simulink subsystem "GS3DX_KDS_Spherical"  (R2025b)
settings: Solver=VariableStepAuto  StartTime=0.0  StopTime=10.0  RelTol=1e-3
model mask{StartPositionX=0, StartPositionY=0, StartPositionZ=0, StartVelocityX=0, StartVelocityY=0, StartVelocityZ=0, DampeningX=0, DampeningY=0, DampeningZ=0, RxPositionTargetPriority=None, RyPositionTargetPriority=None, RzPositionTargetPriority=None, RxVelocityTargetPriority=None, RyVelocityTargetPriority=None, RzVelocityTargetPriority=None}
  mask prompts: StartPositionX "Start Position X (deg)"; StartPositionY "Start Position Y (deg)"; StartPositionZ "Start Position Z (deg)"; StartVelocityX "Start Velocity X (deg/s)"; StartVelocityY "Start Velocity Y (deg/s)"; StartVelocityZ "Start Velocity Z (deg/s)"; DampeningX "Dampening X (Nm/deg/s)"; DampeningY "Dampening Y (Nm/deg/s)"; DampeningZ "Dampening Z (Nm/deg/s)"; RxPositionTargetPriority "Position Target Priority X"; RyPositionTargetPriority "Position Target Priority Y"; RzPositionTargetPriority "Position Target Priority Z"; RxVelocityTargetPriority "Velocity Target Priority X"; RyVelocityTargetPriority "Velocity Target Priority Y"; RzVelocityTargetPriority "Velocity Target Priority Z"
undefined symbols (not defined in the file): DampeningGlobalGain, gs3dx_xyz_rate_matrix, LocalDampeningEnable, X, Y, Z
libraries: nesl_utility x13, sm_lib x3
settings Model: Creator=diete  LastModifiedBy=diete

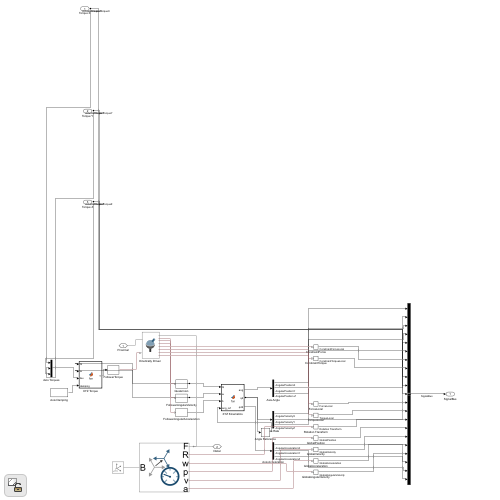
[thumbnail: Simulink's stored preview of the top-level diagram]
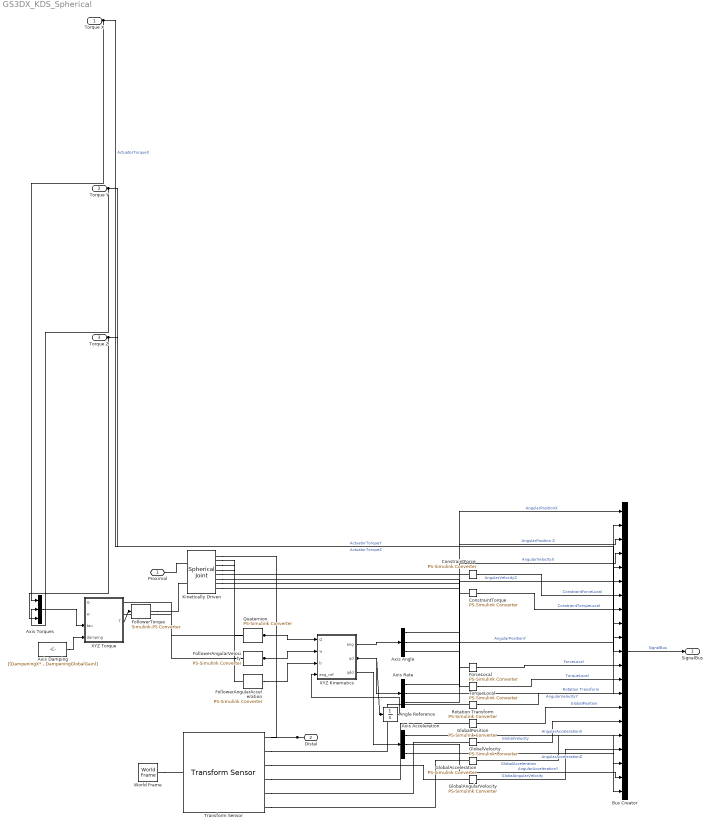
== system GS3DX_KDS_Spherical ==
  Torque X : Inport
  Torque Y : Inport  Port=2
  Torque Z : Inport  Port=3
  Angle Reference : Integrator  InitialCondition=[(StartPositionX); (StartPositionY); (StartPositionZ)]
  Axis Acceleration : Demux  Outputs=3
  Axis Angle : Demux  Outputs=3
  Axis Damping : Constant  Value=[(DampeningX*LocalDampeningEnable*DampeningGlobalGain); (DampeningY*LocalDampeningEnable*DampeningGlobalGain); (DampeningZ*LocalDampeningEnable*DampeningGlobalGain)]  SampleTime=0
  Axis Rate : Demux  Outputs=3
  Axis Torques : Mux  Inputs=3
  Bus Creator : BusCreator  Inputs=21
  ConstraintForce : nesl_utility/PS-Simulink Converter  PhysicalDomain=network_engine_domain  SubClassName=ps_output  LeftPortType=input  RightPortType=output  PseudoPeriodic=off  Frequencies=[]  VectorFormat=1-D array  Unit=inherit  AffineConversion=off
  ConstraintTorque : nesl_utility/PS-Simulink Converter  PhysicalDomain=network_engine_domain  SubClassName=ps_output  LeftPortType=input  RightPortType=output  PseudoPeriodic=off  Frequencies=[]  VectorFormat=1-D array  Unit=inherit  AffineConversion=off
  FollowerAngularAcceleration : nesl_utility/PS-Simulink Converter  PhysicalDomain=network_engine_domain  SubClassName=ps_output  LeftPortType=input  RightPortType=output  PseudoPeriodic=off  Frequencies=[]  VectorFormat=inherit  Unit=rad/s^2  AffineConversion=off
  FollowerAngularVelocity : nesl_utility/PS-Simulink Converter  PhysicalDomain=network_engine_domain  SubClassName=ps_output  LeftPortType=input  RightPortType=output  PseudoPeriodic=off  Frequencies=[]  VectorFormat=inherit  Unit=rad/s  AffineConversion=off
  FollowerTorque : nesl_utility/Simulink-PS Converter  PhysicalDomain=network_engine_domain  SubClassName=ps_input  LeftPortType=input  RightPortType=output  PseudoPeriodic=off  Frequencies=[]  NoiseDistribution=none  NoiseParameters=[]  Unit=N*m  AffineConversion=off  FilteringAndDerivatives=provide  SimscapeFilterOrder=1  InputFilterTimeConstant=0.001  UdotUserProvided=0
  ForceLocal : nesl_utility/PS-Simulink Converter  PhysicalDomain=network_engine_domain  SubClassName=ps_output  LeftPortType=input  RightPortType=output  PseudoPeriodic=off  Frequencies=[]  VectorFormat=1-D array  Unit=inherit  AffineConversion=off
  GlobalAcceleration : nesl_utility/PS-Simulink Converter  PhysicalDomain=network_engine_domain  SubClassName=ps_output  LeftPortType=input  RightPortType=output  PseudoPeriodic=off  Frequencies=[]  VectorFormat=1-D array  Unit=inherit  AffineConversion=off
  GlobalAngularVelocity : nesl_utility/PS-Simulink Converter  PhysicalDomain=network_engine_domain  SubClassName=ps_output  LeftPortType=input  RightPortType=output  PseudoPeriodic=off  Frequencies=[]  VectorFormat=1-D array  Unit=deg/s  AffineConversion=off
  GlobalPosition : nesl_utility/PS-Simulink Converter  PhysicalDomain=network_engine_domain  SubClassName=ps_output  LeftPortType=input  RightPortType=output  PseudoPeriodic=off  Frequencies=[]  VectorFormat=1-D array  Unit=inherit  AffineConversion=off
  GlobalVelocity : nesl_utility/PS-Simulink Converter  PhysicalDomain=network_engine_domain  SubClassName=ps_output  LeftPortType=input  RightPortType=output  PseudoPeriodic=off  Frequencies=[]  VectorFormat=1-D array  Unit=inherit  AffineConversion=off
  Kinetically Driven : sm_lib/Joints/Spherical Joint  JointMode=Normal  CompositeWrenchDir=BaseOnFollower  CompositeWrenchFrame=FollowerFrame  SenseConstraintForce=on  SenseConstraintTorque=on  SenseTotalForce=on  SenseTotalTorque=on  PositionTargetSpecify=off  PositionTargetPriority=High  PositionTargetRotationMethod=RotationSequence  PositionTargetFollAlignAxisA=+X  PositionTargetBaseAlignAxisA=+Y  PositionTargetFollAlignAxisB=+Y  PositionTargetBaseAlignAxisB=+Z  PositionTargetRotationStandardAxis=+Z  PositionTargetRotationAngle=0  PositionTargetRotationAngleUnits=deg  PositionTargetRotationArbitraryAxis=[0 0 1]  PositionTargetRotationSequenceAxes=FollowerAxes  PositionTargetRotationSequence=XYZ  PositionTargetRotationSequenceAngles=[(StartPositionX) (StartPositionY) (StartPositionZ)]  PositionTargetRotationSequenceAnglesUnits=deg  PositionTargetRotationMatrix=[1 0 0;0 1 0;0 0 1]  PositionTargetQuaternion=[1 0 0 0]  VelocityTargetSpecify=off  VelocityTargetPriority=High  VelocityTargetValue=gs3dx_xyz_rate_matrix((StartPositionY)*pi/180, (StartPositionZ)*pi/180)*[(StartVelocityX); (StartVelocityY); (StartVelocityZ)]  VelocityTargetValueUnits=deg/s  VelocityTargetInFollowerFrame=on  EqPosRotationMethod=None  EqPosFollAlignAxisA=+X  EqPosBaseAlignAxisA=+Y  EqPosFollAlignAxisB=+Y  EqPosBaseAlignAxisB=+Z  EqPosRotationStandardAxis=+Z  EqPosRotationAngle=0  EqPosRotationAngleUnits=deg  EqPosRotationArbitraryAxis=[0 0 1]  EqPosRotationSequenceAxes=FollowerAxes  EqPosRotationSequence=XYX  EqPosRotationSequenceAngles=[0 0 0]  EqPosRotationSequenceAnglesUnits=deg  EqPosRotationMatrix=[1 0 0;0 1 0;0 0 1]  EqPosQuaternion=[1 0 0 0]  SpringStiffness=0  SpringStiffnessUnits=N*m/deg  DampingCoefficient=0  DampingCoefficientUnits=N*m/(deg/s)  LowerLimitSpecify=off  LowerLimitBound=15  LowerLimitBoundUnits=deg  LowerLimitStiffness=1e4  LowerLimitStiffnessUnits=N*m/deg  LowerLimitDamping=10  LowerLimitDampingUnits=N*m/(deg/s)  LowerLimitTransitionRegionWidth=0.1  LowerLimitTransitionRegionWidthUnits=deg  UpperLimitSpecify=off  UpperLimitBound=45  UpperLimitBoundUnits=deg  UpperLimitStiffness=1e4  UpperLimitStiffnessUnits=N*m/deg  UpperLimitDamping=10  UpperLimitDampingUnits=N*m/(deg/s)  UpperLimitTransitionRegionWidth=0.1  UpperLimitTransitionRegionWidthUnits=deg  TorqueActuationMode=InputTorque  ActuateTorqueX=off  ActuateTorqueY=off  ActuateTorqueZ=off  ActuateTorque=on  ActuationFrame=FollowerFrame  SensePosition=on  SenseVelocityX=off  SenseVelocityY=off  SenseVelocityZ=off  SenseVelocity=on  SenseAccelerationX=off  SenseAccelerationY=off  SenseAccelerationZ=off  SenseAcceleration=on  SenseLowerLimitTorqueMag=off  SenseUpperLimitTorqueMag=off  SensingFrame=FollowerFrame
  Quaternion : nesl_utility/PS-Simulink Converter  PhysicalDomain=network_engine_domain  SubClassName=ps_output  LeftPortType=input  RightPortType=output  PseudoPeriodic=off  Frequencies=[]  VectorFormat=inherit  Unit=1  AffineConversion=off
  Rotation Transform : nesl_utility/PS-Simulink Converter  PhysicalDomain=network_engine_domain  SubClassName=ps_output  LeftPortType=input  RightPortType=output  PseudoPeriodic=off  Frequencies=[]  VectorFormat=1-D array  Unit=inherit  AffineConversion=off
  TorqueLocal : nesl_utility/PS-Simulink Converter  PhysicalDomain=network_engine_domain  SubClassName=ps_output  LeftPortType=input  RightPortType=output  PseudoPeriodic=off  Frequencies=[]  VectorFormat=1-D array  Unit=inherit  AffineConversion=off
  Transform Sensor : sm_lib/Frames and Transforms/Transform Sensor  MeasurementFrame=World  RotationSequence=XYX  SenseAngle=off  SenseAxis=off  SenseQ=off  SenseR=on  SenseRotationSequence=off  SenseOmegaX=off  SenseOmegaY=off  SenseOmegaZ=off  SenseOmega=on  SenseQDot=off  SenseRDot=off  SenseRotationSequenceDot=off  SenseAlphaX=off  SenseAlphaY=off  SenseAlphaZ=off  SenseAlpha=off  SenseQDDot=off  SenseRDDot=off  SenseX=off  SenseY=off  SenseZ=off  SenseXYZ=on  SenseRad=off  SenseAzim=off  SenseDist=off  SenseInc=off  SenseXDot=off  SenseYDot=off  SenseZDot=off  SenseXYZDot=on  SenseRadDot=off  SenseAzimDot=off  SenseDistDot=off  SenseIncDot=off  SenseXDDot=off  SenseYDDot=off  SenseZDDot=off  SenseXYZDDot=on  SenseRadDDot=off  SenseAzimDDot=off  SenseDistDDot=off  SenseIncDDot=off
  World Frame : sm_lib/Frames and Transforms/World Frame
  XYZ Kinematics : MATLAB Function  TreatAsAtomicUnit=on
  XYZ Torque : MATLAB Function  TreatAsAtomicUnit=on
  Proximal : PMIOPort  Side=Left
  Distal : PMIOPort  Port=2  Side=Right
  SignalBus : Outport
  wires:
  Rotation Transform/1 -> Bus Creator/14  "Rotation Transform"
  ForceLocal/1 -> Bus Creator/12  "ForceLocal"
  ConstraintTorque/1 -> Bus Creator/8  "ConstraintTorqueLocal"
  GlobalAcceleration/1 -> Bus Creator/17  "GlobalAcceleration"
  GlobalAngularVelocity/1 -> Bus Creator/18  "GlobalAngularVelocity"
  ConstraintForce/1 -> Bus Creator/7  "ConstraintForceLocal"
  TorqueLocal/1 -> Bus Creator/13  "TorqueLocal"
  GlobalVelocity/1 -> Bus Creator/16  "GlobalVelocity"
  GlobalPosition/1 -> Bus Creator/15  "GlobalPosition"
  Bus Creator/1 -> SignalBus/1  "SignalBus"
  Torque X/1 -> Axis Torques/1, Bus Creator/9  "ActuatorTorqueX"
  Torque Y/1 -> Axis Torques/2, Bus Creator/10  "ActuatorTorqueY"
  Torque Z/1 -> Axis Torques/3, Bus Creator/11  "ActuatorTorqueZ"
  Quaternion/1 -> XYZ Torque/1(Q), XYZ Kinematics/1(Q)
  FollowerAngularVelocity/1 -> XYZ Torque/2(w), XYZ Kinematics/2(w)
  Axis Torques/1 -> XYZ Torque/3(tau)
  Axis Damping/1 -> XYZ Torque/4(damping)
  XYZ Torque/1(T) -> FollowerTorque/1
  FollowerAngularAcceleration/1 -> XYZ Kinematics/3(b)
  Angle Reference/1 -> XYZ Kinematics/4(ang_ref)
  XYZ Kinematics/2(qd) -> Angle Reference/1, Axis Rate/1
  XYZ Kinematics/1(ang) -> Axis Angle/1
  Axis Angle/1 -> Bus Creator/1  "AngularPositionX"
  Axis Angle/2 -> Bus Creator/2  "AngularPositionY"
  Axis Angle/3 -> Bus Creator/3  "AngularPosition Z"
  Axis Rate/1 -> Bus Creator/4  "AngularVelocityX"
  Axis Rate/2 -> Bus Creator/5  "AngularVelocityY"
  Axis Rate/3 -> Bus Creator/6  "AngularVelocityZ"
  XYZ Kinematics/3(qdd) -> Axis Acceleration/1
  Axis Acceleration/1 -> Bus Creator/19  "AngularAccelerationX"
  Axis Acceleration/2 -> Bus Creator/20  "AngularAccelerationY"
  Axis Acceleration/3 -> Bus Creator/21  "AngularAccelerationZ"
  connections:
  Transform Sensor/RConn4 -- GlobalPosition/LConn1
  Transform Sensor/RConn2 -- Rotation Transform/LConn1
  Transform Sensor/RConn3 -- GlobalAngularVelocity/LConn1
  Transform Sensor/RConn6 -- GlobalAcceleration/LConn1
  Transform Sensor/RConn5 -- GlobalVelocity/LConn1
  World Frame/RConn1 -- Transform Sensor/LConn1
  Distal/RConn1 -- Transform Sensor/RConn1 -- Kinetically Driven/RConn1
  Kinetically Driven/LConn1 -- Proximal/RConn1
  Kinetically Driven/RConn5 -- ConstraintForce/LConn1
  Kinetically Driven/RConn6 -- ConstraintTorque/LConn1
  Kinetically Driven/RConn7 -- ForceLocal/LConn1
  Kinetically Driven/RConn8 -- TorqueLocal/LConn1
  FollowerTorque/RConn1 -- Kinetically Driven/LConn2
  Kinetically Driven/RConn2 -- Quaternion/LConn1
  Kinetically Driven/RConn3 -- FollowerAngularVelocity/LConn1
  Kinetically Driven/RConn4 -- FollowerAngularAcceleration/LConn1

== matlab function GS3DX_KDS_Spherical/XYZ Kinematics ==
  data: Q input; ang output; w input; b input; ang_ref input; qd output; qdd output
function [ang, qd, qdd] = fcn(Q, w, b, ang_ref)
% Quaternion state -> X-Y-Z angles, rates, accelerations (deg).
[~, ang, qd, qdd] = gs3dx_xyz_map(Q, w, b, zeros(3, 1), zeros(3, 1), ang_ref);

== matlab function GS3DX_KDS_Spherical/XYZ Torque ==
  data: Q input; T output; w input; tau input; damping input
function T = fcn(Q, w, tau, damping)
% Axis torques -> follower-frame torque (gs3dx_xyz_map).
T = gs3dx_xyz_map(Q, w, zeros(3, 1), tau, damping, zeros(3, 1));
